simulink model "simulink_seance32"  (R2013b)
settings: Solver=FixedStepDiscrete  StartTime=0.0  StopTime=Tf  FixedStep=Te  RelTol=1e-3
undefined symbols (not defined in the file): Ka, Kb, Te
settings Model: TunableVars=Ka,Kb,Kd,Te  TunableVarsStorageClass=Auto,Auto,Auto,Auto  TunableVarsTypeQualifier=,,,  Creator=gemsdev  LastModifiedBy=gemsdev
settings DataIOCC: LoadExternalInput=on
settings OptimizationCC: InlineParams=on  OptimizeModelRefInitCode=on  LifeSpan=1
settings RTWCC: SystemTargetFile=ert.tlc  TemplateMakefile=RTW.MSVCBuild  Description=Create Visual C/C++ Solution File for Embedded Coder  ProcessScript=ert_make_rtw_hook  TargetLang=C++
settings CodeAppCC: IgnoreCustomStorageClasses=off
settings ERTTargetCC: CodeReplacementLibrary=ANSI_C  GenerateSampleERTMain=on  InlinedParameterPlacement=NonHierarchical  ERTCustomFileTemplate=example_file_process.tlc

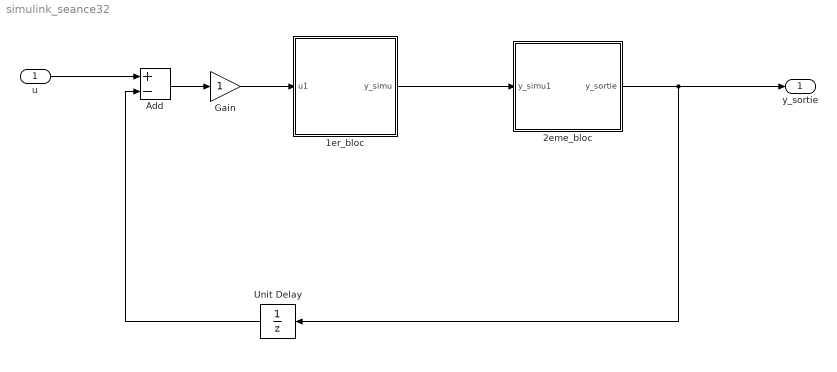
== system simulink_seance32 ==
  u : Inport
  1er_bloc : Subsystem
  2eme_bloc : Subsystem
  Add : Sum  Inputs=+-
  Gain : Gain
  Unit Delay : UnitDelay  SampleTime=-1
  y_sortie : Outport
  wires:
  2eme_bloc/1(y_sortie) -> Unit Delay/1, y_sortie/1
  1er_bloc/1(y_simu) -> 2eme_bloc/1(y_simu1)
  u/1 -> Add/1
  Add/1 -> Gain/1
  Unit Delay/1 -> Add/2
  Gain/1 -> 1er_bloc/1(u1)

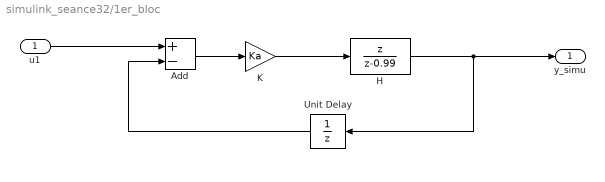
== system simulink_seance32/1er_bloc ==
  u1 : Inport
  Add : Sum  Inputs=+-  SampleTime=Te
  H : DiscreteTransferFcn  Numerator=[1 0]  Denominator=[1 -0.99]  SampleTime=Te
  K : Gain  Gain=Ka  SampleTime=Te
  Unit Delay : UnitDelay  SampleTime=Te
  y_simu : Outport
  wires:
  Add/1 -> K/1
  K/1 -> H/1
  H/1 -> y_simu/1, Unit Delay/1
  Unit Delay/1 -> Add/2
  u1/1 -> Add/1

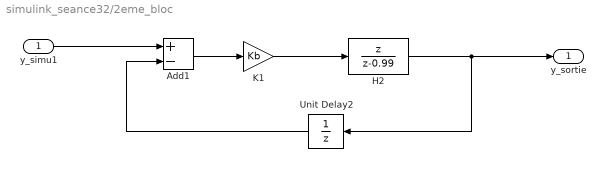
== system simulink_seance32/2eme_bloc ==
  y_simu1 : Inport
  Add1 : Sum  Inputs=+-  SampleTime=Te
  H2 : DiscreteTransferFcn  Numerator=[1 0]  Denominator=[1 -0.99]  SampleTime=Te
  K1 : Gain  Gain=Kb  SampleTime=Te
  Unit Delay2 : UnitDelay  SampleTime=Te
  y_sortie : Outport
  wires:
  y_simu1/1 -> Add1/1
  H2/1 -> y_sortie/1, Unit Delay2/1
  Add1/1 -> K1/1
  Unit Delay2/1 -> Add1/2
  K1/1 -> H2/1
